simulink model "pwmGenerator"  (R2014b)
settings: Solver=ode45  StartTime=0.0  StopTime=10.0  RelTol=1e-3
libraries: simulink x1

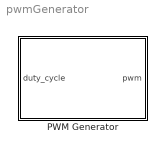
== system pwmGenerator ==
  PWM Generator : Subsystem  mask{pwmResolution=0, pwmClockPeriod=0}
      mask prompts: pwmResolution "PWM Resultion [bits]"; pwmClockPeriod "PWM Clock Period [s]"
      mask help:
      | The resolution of the duty cycle between 0 and 1 is calculated as 1/(2^pwmResolution)
      | The frequency [Hz] of the pwm signal is determined by 1/(2^pwmResolution*pwmClockPeriod)
      |
      | Inside the PWM generate is a counter and a comparator. The counter increments its value by 1 for every PWM clock period and resets to zero after reaching its maximum value deterined by the number of bits of resolution.
      |
      | This creates a trade off between high duty cycle resultion and a high pwm clock frequency.

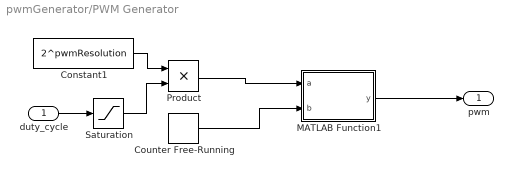
== system pwmGenerator/PWM Generator ==
  duty_cycle : Inport
  Constant1 : Constant  Value=2^pwmResolution
  Counter Free-Running : simulink/Sources/Counter Free-Running  NumBits=pwmResolution  tsamp=pwmClockPeriod
  MATLAB Function1 : MATLAB Function  TreatAsAtomicUnit=on
      mask help: y = (a >= b) ? 1 : 0;
  Product : Product
  Saturation : Saturate  UpperLimit=1  LowerLimit=0
  pwm : Outport
  wires:
  MATLAB Function1/1(y) -> pwm/1
  Product/1 -> MATLAB Function1/1(a)
  Constant1/1 -> Product/1
  Counter Free-Running/1 -> MATLAB Function1/2(b)
  Saturation/1 -> Product/2
  duty_cycle/1 -> Saturation/1

== matlab function pwmGenerator/PWM Generator/MATLAB Function1 ==
function y = Comparator(a, b)
    if a>= b
        y = 1;
    else
        y = 0;
    end
